simulink model "model_stabilizer_only"  (R2022b)
settings: Solver=VariableStepAuto  StartTime=0.0  StopTime=20  MaxStep=0.1  RelTol=1e-3
libraries: cstblocks x6
settings Model: Creator=mohammadmahdi  LastModifiedBy=Alireza
settings ModelReferenceCC: EnableRefExpFcnMdlSchedulingChecks=on

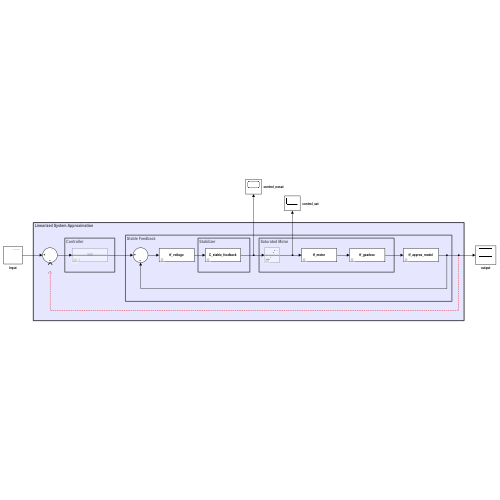
[thumbnail: Simulink's stored preview of the top-level diagram]
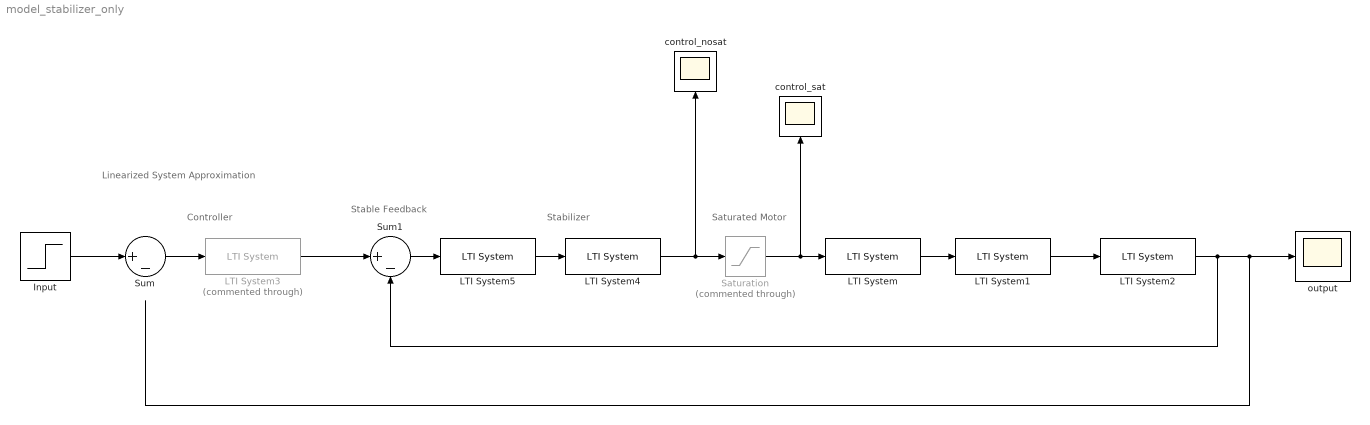
== system model_stabilizer_only ==
  note: Stable Feedback
  note: Linearized System Approximation
  note: Controller
  note: Stabilizer
  note: Saturated Motor
  Input : Step  After=0.5  SampleTime=0
  LTI System : cstblocks/LTI System  sys=tf_motor  IC=[]
  LTI System1 : cstblocks/LTI System  sys=tf_gearbox  IC=[]
  LTI System2 : cstblocks/LTI System  sys=tf_approx_model  IC=[]
  LTI System3 : cstblocks/LTI System  Commented=through  sys=tf_controller  IC=[]
  LTI System4 : cstblocks/LTI System  sys=C_stable_feedback  IC=[]
  LTI System5 : cstblocks/LTI System  sys=tf_voltage  IC=[]
  Saturation : Saturate  Commented=through  UpperLimit=15  LowerLimit=-15
  Sum : Sum  Inputs=|+-
  Sum1 : Sum  Inputs=|+-
  control_nosat : Scope
  control_sat : Scope
  output : Scope
  wires:
  Sum/1 -> LTI System3/1
  Input/1 -> Sum/1
  LTI System4/1 -> control_nosat/1, Saturation/1
  Saturation/1 -> LTI System/1, control_sat/1
  LTI System1/1 -> LTI System2/1
  LTI System2/1 -> Sum1/2, output/1
  LTI System3/1 -> Sum1/1
  LTI System/1 -> LTI System1/1
  LTI System5/1 -> LTI System4/1
  Sum1/1 -> LTI System5/1
